simulink model "Full_Motor_Sim"  (R2020b)
settings: Solver=VariableStepAuto  StartTime=0.0  StopTime=1  RelTol=1e-3
libraries: fl_lib x26, ee_lib x20, nesl_utility x19, simulink x12
(part 2 of 2)

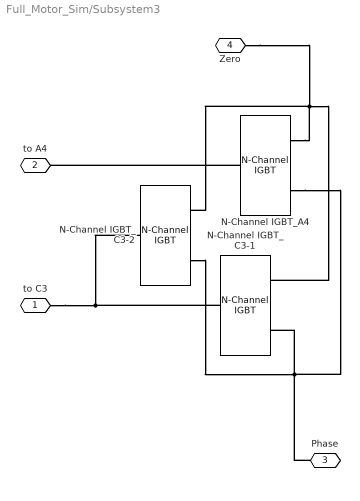
== system Full_Motor_Sim/Subsystem3 ==
  N-Channel IGBT_A4 : ee_lib/Semiconductors & Converters/N-Channel IGBT  model_type=1  Ices=25 uA  Vces=1200 V  Vth=5 V  Vce_sat=1.4 V  Ice_sat=110 A  Vge_sat=15 V  ec=1.3  Tmeas=25 degC  Vge_vec=[ -2 6 7 8 10 12 15 20 ] V  Vce_vec=[ -1 0 0.5 1 1.5 2 2.5 3 3.5 4 ] V  T_vec=[25, 125] degC  Ic_mat=[ -1.015e-5 1.35e-8 4.7135e-4 5.092e-4 5.105e-4 5.117500000000001e-4 5.1299e-4 5.1423e-4 5.1548e-4 5.1672e-4; -9.986899999999999e-6 1.35e-8 4.7135e-4 5.092e-4 5.105e-4 5.117500000000001e-4 5.1299e-4 5.1423e-4 5.1548e-4 5.1672e-4; -9.955e-6 1.35e-8 0.0065225 3.3324 48.154 93.661 105.52 105.72 105.93 106.14; -9.955e-6 1.35e-8 0.0065235 3.5783 70.264 166.33 252.4 317.67 353.38 357.39; -9.955e-6 1.35e-8 0.006524 3.7206 89.17100000000001 228.09 371.63 511.02 642.6900000000001 764.04; -9.9549e-6 1.35e-8 0.0065242 3.7716 97.79300000000001 256.21 424.27 592.92 759.2 921.52; -9.9549e-6 1.35e-8 0.0065243 3.8067 104.52 278.11 464.6 654.37 844.5700000000001 1.0339e+3; -9.9549e-6 1.35e-8 0.0065244 3.8324 109.92 295.67 496.54 702.28 909.96 1.1183e+3 ] A  Ic_mat_3D=zeros(8, 10, 2) A  C_param=3  C_GE=23.7 nF  C_GC=2.7 nF  C_CE=0 nF  C_ies=9.85 nF  C_res=218 pF  C_oes=580 pF  C_GE_vec=[ 25 31 26.5 24.9 25 24.9 24.6 24.7 24.8 ] nF  C_GC_vec=[ 55 9 5.5 3.1 2.5 2.1 1.9 1.8 1.7 ] nF  C_CE_vec=[ 5 11 6.5 4.9 3.5 2.7 2.1 1.7 1.4 ] nF  C_ies_vec=[70 62 60 60 60 60 60 60 60 ] nF  C_res_vec=[ 12 0.46 0.32 0.28 0.24 0.22 0.2 0.19 0.16 ] nF  C_oes_vec=[ 31 0.73 0.515 0.44 0.38 0.34 0.31 0.29 0.28 ] nF  C_Vce_vec=[ 0 5 10 15 20 25 30 35 40 ] V  charge_linearity_param=1  C_OX=20 nF  V_C_OX=-5 V  TF=0 ns  VAF=350 V  RC=0.0001 Ohm  RE=0.0045 Ohm  RG=1 Ohm  BF=100  T_param=2  Ices_T2=620 uA  EG=0.0001 eV  Vce_sat_T2=1.6 V  Tmeas2=150 degC  XTI=1  BEX=-0.6  RG_alpha=1 1/K  Tdevice=150 degC  Tdevice_3D=25 degC  thermal_network_parameterization=ee.enum.thermalNetworkTopology.cauer  Rth=[0, 10] K/W  Rth_Foster=[4, 6] K/W  thermal_mass_parameterization=ee.enum.thermalNetwork.timeconstant  thermal_mass=[0, 1] J/K  thermal_mass_Foster=[1.5, 3] J/K  thermal_time_constant=[0, 10] s  thermal_time_constant_Foster=[6, 18] s  thermal_mass_initial_temperatures=[25, 25] degC  Ic_vec1=[0, 10, 50, 100, 200, 400, 600] A  Vce_vec1=[0, 1.1, 1.3, 1.45, 1.75, 2.25, 2.7] V  Rmiller=0.1 Ohm  Goff=1e-5 1/Ohm  t_on=0.07 us  t_rise=0.7 us  t_off=0.2 us  t_fall=0.5 us  v_meas=300 V  Tj_vec1=[298.15, 398.15] K  Vce_mat1=[0, 1.1, 1.3, 1.45, 1.75, 2.25, 2.7; 0, 1, 1.15, 1.35, 1.7, 2.35, 3] V  E_turn_on_mat1=[0, .2, 1, 2, 4, 8, 15; 0, .3, 1.3, 2.5, 5, 11, 18] * 1e-3 J  E_turn_off_mat1=[0, .3, 1.5, 3, 6, 15, 25; 0, .7, 3.3, 6.5, 13, 25, 35] * 1e-3 J
      settings: SourceProductBaseCode=PS  InternalSimscapePortConfiguration="{\"Bottom\":[],\"Left\":[{\"id\":\"G\",\"label\":\"\",\"type\":\"foundation.electrical.electrical\"}],\"Right\":[{\"id\":\"C\",\"label\":\"\",\"type\":\"foundation.electrical.electrical\"},{\"id\":\"E\",\"label\":\"\",\"type\":\"foundation.electrical.electrical\"}],\"Top\":[]}"
  N-Channel IGBT_C3-1 : ee_lib/Semiconductors & Converters/N-Channel IGBT  model_type=1  Ices=25 uA  Vces=1200 V  Vth=5 V  Vce_sat=2.25 V  Ice_sat=40 A  Vge_sat=7 V  ec=1.5  Tmeas=25 degC  Vge_vec=[ -2 6 7 8 10 12 15 20 ] V  Vce_vec=[ -1 0 0.5 1 1.5 2 2.5 3 3.5 4 ] V  T_vec=[25, 125] degC  Ic_mat=[ -1.015e-5 1.35e-8 4.7135e-4 5.092e-4 5.105e-4 5.117500000000001e-4 5.1299e-4 5.1423e-4 5.1548e-4 5.1672e-4; -9.986899999999999e-6 1.35e-8 4.7135e-4 5.092e-4 5.105e-4 5.117500000000001e-4 5.1299e-4 5.1423e-4 5.1548e-4 5.1672e-4; -9.955e-6 1.35e-8 0.0065225 3.3324 48.154 93.661 105.52 105.72 105.93 106.14; -9.955e-6 1.35e-8 0.0065235 3.5783 70.264 166.33 252.4 317.67 353.38 357.39; -9.955e-6 1.35e-8 0.006524 3.7206 89.17100000000001 228.09 371.63 511.02 642.6900000000001 764.04; -9.9549e-6 1.35e-8 0.0065242 3.7716 97.79300000000001 256.21 424.27 592.92 759.2 921.52; -9.9549e-6 1.35e-8 0.0065243 3.8067 104.52 278.11 464.6 654.37 844.5700000000001 1.0339e+3; -9.9549e-6 1.35e-8 0.0065244 3.8324 109.92 295.67 496.54 702.28 909.96 1.1183e+3 ] A  Ic_mat_3D=zeros(8, 10, 2) A  C_param=3  C_GE=23.7 nF  C_GC=2.7 nF  C_CE=0 nF  C_ies=9.85 nF  C_res=218 pF  C_oes=580 pF  C_GE_vec=[ 25 31 26.5 24.9 25 24.9 24.6 24.7 24.8 ] nF  C_GC_vec=[ 55 9 5.5 3.1 2.5 2.1 1.9 1.8 1.7 ] nF  C_CE_vec=[ 5 11 6.5 4.9 3.5 2.7 2.1 1.7 1.4 ] nF  C_ies_vec=[ 18 13 12 11 10 10 10 10 10 ] nF  C_res_vec=[ 6 2.7 1.9 1.3 0.36 0.22 0.19 0.17 0.16 ] nF  C_oes_vec=[ 8.5 4 3 2 0.8 0.6 0.5 0.48 0.43 ] nF  C_Vce_vec=[ 0 5 10 15 20 25 30 35 40 ] V  charge_linearity_param=1  C_OX=20 nF  V_C_OX=-5 V  TF=0 ns  VAF=10 V  RC=0.005 Ohm  RE=0.009 Ohm  RG=1 kOhm  BF=100  T_param=2  Ices_T2=1.5 mA  EG=0.0001 eV  Vce_sat_T2=2.45 V  Tmeas2=150 degC  XTI=1  BEX=-1  RG_alpha=1 1/K  Tdevice=150 degC  Tdevice_3D=25 degC  thermal_network_parameterization=ee.enum.thermalNetworkTopology.cauer  Rth=[0, 10] K/W  Rth_Foster=[4, 6] K/W  thermal_mass_parameterization=ee.enum.thermalNetwork.timeconstant  thermal_mass=[0, 1] J/K  thermal_mass_Foster=[1.5, 3] J/K  thermal_time_constant=[0, 10] s  thermal_time_constant_Foster=[6, 18] s  thermal_mass_initial_temperatures=[25, 25] degC  Ic_vec1=[0, 10, 50, 100, 200, 400, 600] A  Vce_vec1=[0, 1.1, 1.3, 1.45, 1.75, 2.25, 2.7] V  Rmiller=0.1 Ohm  Goff=1e-5 1/Ohm  t_on=0.07 us  t_rise=0.7 us  t_off=0.2 us  t_fall=0.5 us  v_meas=300 V  Tj_vec1=[298.15, 398.15] K  Vce_mat1=[0, 1.1, 1.3, 1.45, 1.75, 2.25, 2.7; 0, 1, 1.15, 1.35, 1.7, 2.35, 3] V  E_turn_on_mat1=[0, .2, 1, 2, 4, 8, 15; 0, .3, 1.3, 2.5, 5, 11, 18] * 1e-3 J  E_turn_off_mat1=[0, .3, 1.5, 3, 6, 15, 25; 0, .7, 3.3, 6.5, 13, 25, 35] * 1e-3 J
      settings: SourceProductName=Electrical  InternalSimscapePortConfiguration="{\"Bottom\":[],\"Left\":[{\"id\":\"G\",\"label\":\"\",\"type\":\"foundation.electrical.electrical\"}],\"Right\":[{\"id\":\"C\",\"label\":\"\",\"type\":\"foundation.electrical.electrical\"},{\"id\":\"E\",\"label\":\"\",\"type\":\"foundation.electrical.electrical\"}],\"Top\":[]}"
  N-Channel IGBT_C3-2 : ee_lib/Semiconductors & Converters/N-Channel IGBT  model_type=1  Ices=25 uA  Vces=1200 V  Vth=5 V  Vce_sat=2.25 V  Ice_sat=40 A  Vge_sat=7 V  ec=1.5  Tmeas=25 degC  Vge_vec=[ -2 6 7 8 10 12 15 20 ] V  Vce_vec=[ -1 0 0.5 1 1.5 2 2.5 3 3.5 4 ] V  T_vec=[25, 125] degC  Ic_mat=[ -1.015e-5 1.35e-8 4.7135e-4 5.092e-4 5.105e-4 5.117500000000001e-4 5.1299e-4 5.1423e-4 5.1548e-4 5.1672e-4; -9.986899999999999e-6 1.35e-8 4.7135e-4 5.092e-4 5.105e-4 5.117500000000001e-4 5.1299e-4 5.1423e-4 5.1548e-4 5.1672e-4; -9.955e-6 1.35e-8 0.0065225 3.3324 48.154 93.661 105.52 105.72 105.93 106.14; -9.955e-6 1.35e-8 0.0065235 3.5783 70.264 166.33 252.4 317.67 353.38 357.39; -9.955e-6 1.35e-8 0.006524 3.7206 89.17100000000001 228.09 371.63 511.02 642.6900000000001 764.04; -9.9549e-6 1.35e-8 0.0065242 3.7716 97.79300000000001 256.21 424.27 592.92 759.2 921.52; -9.9549e-6 1.35e-8 0.0065243 3.8067 104.52 278.11 464.6 654.37 844.5700000000001 1.0339e+3; -9.9549e-6 1.35e-8 0.0065244 3.8324 109.92 295.67 496.54 702.28 909.96 1.1183e+3 ] A  Ic_mat_3D=zeros(8, 10, 2) A  C_param=3  C_GE=23.7 nF  C_GC=2.7 nF  C_CE=0 nF  C_ies=9.85 nF  C_res=218 pF  C_oes=580 pF  C_GE_vec=[ 25 31 26.5 24.9 25 24.9 24.6 24.7 24.8 ] nF  C_GC_vec=[ 55 9 5.5 3.1 2.5 2.1 1.9 1.8 1.7 ] nF  C_CE_vec=[ 5 11 6.5 4.9 3.5 2.7 2.1 1.7 1.4 ] nF  C_ies_vec=[ 18 13 12 11 10 10 10 10 10 ] nF  C_res_vec=[ 6 2.7 1.9 1.3 0.36 0.22 0.19 0.17 0.16 ] nF  C_oes_vec=[ 8.5 4 3 2 0.8 0.6 0.5 0.48 0.43 ] nF  C_Vce_vec=[ 0 5 10 15 20 25 30 35 40 ] V  charge_linearity_param=1  C_OX=20 nF  V_C_OX=-5 V  TF=0 ns  VAF=10 V  RC=0.005 Ohm  RE=0.009 Ohm  RG=1 kOhm  BF=100  T_param=2  Ices_T2=1.5 mA  EG=0.0001 eV  Vce_sat_T2=2.45 V  Tmeas2=150 degC  XTI=1  BEX=-1  RG_alpha=1 1/K  Tdevice=150 degC  Tdevice_3D=25 degC  thermal_network_parameterization=ee.enum.thermalNetworkTopology.cauer  Rth=[0, 10] K/W  Rth_Foster=[4, 6] K/W  thermal_mass_parameterization=ee.enum.thermalNetwork.timeconstant  thermal_mass=[0, 1] J/K  thermal_mass_Foster=[1.5, 3] J/K  thermal_time_constant=[0, 10] s  thermal_time_constant_Foster=[6, 18] s  thermal_mass_initial_temperatures=[25, 25] degC  Ic_vec1=[0, 10, 50, 100, 200, 400, 600] A  Vce_vec1=[0, 1.1, 1.3, 1.45, 1.75, 2.25, 2.7] V  Rmiller=0.1 Ohm  Goff=1e-5 1/Ohm  t_on=0.07 us  t_rise=0.7 us  t_off=0.2 us  t_fall=0.5 us  v_meas=300 V  Tj_vec1=[298.15, 398.15] K  Vce_mat1=[0, 1.1, 1.3, 1.45, 1.75, 2.25, 2.7; 0, 1, 1.15, 1.35, 1.7, 2.35, 3] V  E_turn_on_mat1=[0, .2, 1, 2, 4, 8, 15; 0, .3, 1.3, 2.5, 5, 11, 18] * 1e-3 J  E_turn_off_mat1=[0, .3, 1.5, 3, 6, 15, 25; 0, .7, 3.3, 6.5, 13, 25, 35] * 1e-3 J
      settings: SourceProductName=Electrical  InternalSimscapePortConfiguration="{\"Bottom\":[],\"Left\":[{\"id\":\"G\",\"label\":\"\",\"type\":\"foundation.electrical.electrical\"}],\"Right\":[{\"id\":\"C\",\"label\":\"\",\"type\":\"foundation.electrical.electrical\"},{\"id\":\"E\",\"label\":\"\",\"type\":\"foundation.electrical.electrical\"}],\"Top\":[]}"
  to C3 : PMIOPort  Side=Left
  to A4 : PMIOPort  Port=2  Side=Left
  Phase : PMIOPort  Port=3  Side=Left
  Zero : PMIOPort  Port=4  Side=Right
  connections:
  N-Channel IGBT_A4/LConn1 -- to A4/RConn1
  Phase/RConn1 -- N-Channel IGBT_C3-2/RConn1 -- N-Channel IGBT_A4/RConn1 -- N-Channel IGBT_C3-1/RConn1
  Zero/RConn1 -- N-Channel IGBT_C3-1/RConn2 -- N-Channel IGBT_A4/RConn2 -- N-Channel IGBT_C3-2/RConn2
  N-Channel IGBT_C3-1/LConn1 -- to C3/RConn1 -- N-Channel IGBT_C3-2/LConn1

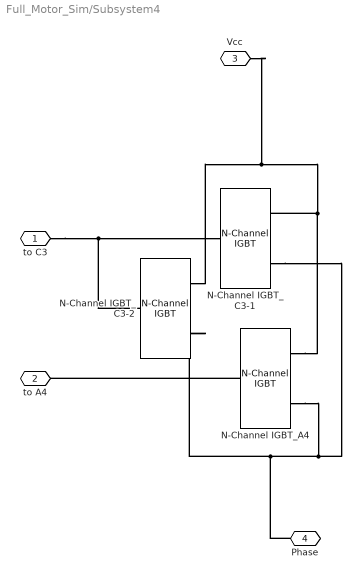
== system Full_Motor_Sim/Subsystem4 ==
  N-Channel IGBT_A4 : ee_lib/Semiconductors & Converters/N-Channel IGBT  model_type=1  Ices=25 uA  Vces=1200 V  Vth=5 V  Vce_sat=1.4 V  Ice_sat=110 A  Vge_sat=15 V  ec=1.3  Tmeas=25 degC  Vge_vec=[ -2 6 7 8 10 12 15 20 ] V  Vce_vec=[ -1 0 0.5 1 1.5 2 2.5 3 3.5 4 ] V  T_vec=[25, 125] degC  Ic_mat=[ -1.015e-5 1.35e-8 4.7135e-4 5.092e-4 5.105e-4 5.117500000000001e-4 5.1299e-4 5.1423e-4 5.1548e-4 5.1672e-4; -9.986899999999999e-6 1.35e-8 4.7135e-4 5.092e-4 5.105e-4 5.117500000000001e-4 5.1299e-4 5.1423e-4 5.1548e-4 5.1672e-4; -9.955e-6 1.35e-8 0.0065225 3.3324 48.154 93.661 105.52 105.72 105.93 106.14; -9.955e-6 1.35e-8 0.0065235 3.5783 70.264 166.33 252.4 317.67 353.38 357.39; -9.955e-6 1.35e-8 0.006524 3.7206 89.17100000000001 228.09 371.63 511.02 642.6900000000001 764.04; -9.9549e-6 1.35e-8 0.0065242 3.7716 97.79300000000001 256.21 424.27 592.92 759.2 921.52; -9.9549e-6 1.35e-8 0.0065243 3.8067 104.52 278.11 464.6 654.37 844.5700000000001 1.0339e+3; -9.9549e-6 1.35e-8 0.0065244 3.8324 109.92 295.67 496.54 702.28 909.96 1.1183e+3 ] A  Ic_mat_3D=zeros(8, 10, 2) A  C_param=3  C_GE=23.7 nF  C_GC=2.7 nF  C_CE=0 nF  C_ies=9.85 nF  C_res=218 pF  C_oes=580 pF  C_GE_vec=[ 25 31 26.5 24.9 25 24.9 24.6 24.7 24.8 ] nF  C_GC_vec=[ 55 9 5.5 3.1 2.5 2.1 1.9 1.8 1.7 ] nF  C_CE_vec=[ 5 11 6.5 4.9 3.5 2.7 2.1 1.7 1.4 ] nF  C_ies_vec=[70 62 60 60 60 60 60 60 60 ] nF  C_res_vec=[ 12 0.46 0.32 0.28 0.24 0.22 0.2 0.19 0.16 ] nF  C_oes_vec=[ 31 0.73 0.515 0.44 0.38 0.34 0.31 0.29 0.28 ] nF  C_Vce_vec=[ 0 5 10 15 20 25 30 35 40 ] V  charge_linearity_param=1  C_OX=20 nF  V_C_OX=-5 V  TF=0 ns  VAF=350 V  RC=0.0001 Ohm  RE=0.0045 Ohm  RG=1 Ohm  BF=100  T_param=2  Ices_T2=620 uA  EG=0.0001 eV  Vce_sat_T2=1.6 V  Tmeas2=150 degC  XTI=1  BEX=-0.6  RG_alpha=1 1/K  Tdevice=150 degC  Tdevice_3D=25 degC  thermal_network_parameterization=ee.enum.thermalNetworkTopology.cauer  Rth=[0, 10] K/W  Rth_Foster=[4, 6] K/W  thermal_mass_parameterization=ee.enum.thermalNetwork.timeconstant  thermal_mass=[0, 1] J/K  thermal_mass_Foster=[1.5, 3] J/K  thermal_time_constant=[0, 10] s  thermal_time_constant_Foster=[6, 18] s  thermal_mass_initial_temperatures=[25, 25] degC  Ic_vec1=[0, 10, 50, 100, 200, 400, 600] A  Vce_vec1=[0, 1.1, 1.3, 1.45, 1.75, 2.25, 2.7] V  Rmiller=0.1 Ohm  Goff=1e-5 1/Ohm  t_on=0.07 us  t_rise=0.7 us  t_off=0.2 us  t_fall=0.5 us  v_meas=300 V  Tj_vec1=[298.15, 398.15] K  Vce_mat1=[0, 1.1, 1.3, 1.45, 1.75, 2.25, 2.7; 0, 1, 1.15, 1.35, 1.7, 2.35, 3] V  E_turn_on_mat1=[0, .2, 1, 2, 4, 8, 15; 0, .3, 1.3, 2.5, 5, 11, 18] * 1e-3 J  E_turn_off_mat1=[0, .3, 1.5, 3, 6, 15, 25; 0, .7, 3.3, 6.5, 13, 25, 35] * 1e-3 J
      settings: SourceProductBaseCode=PS  InternalSimscapePortConfiguration="{\"Bottom\":[],\"Left\":[{\"id\":\"G\",\"label\":\"\",\"type\":\"foundation.electrical.electrical\"}],\"Right\":[{\"id\":\"C\",\"label\":\"\",\"type\":\"foundation.electrical.electrical\"},{\"id\":\"E\",\"label\":\"\",\"type\":\"foundation.electrical.electrical\"}],\"Top\":[]}"
  N-Channel IGBT_C3-1 : ee_lib/Semiconductors & Converters/N-Channel IGBT  model_type=1  Ices=25 uA  Vces=1200 V  Vth=5 V  Vce_sat=2.25 V  Ice_sat=40 A  Vge_sat=7 V  ec=1.5  Tmeas=25 degC  Vge_vec=[ -2 6 7 8 10 12 15 20 ] V  Vce_vec=[ -1 0 0.5 1 1.5 2 2.5 3 3.5 4 ] V  T_vec=[25, 125] degC  Ic_mat=[ -1.015e-5 1.35e-8 4.7135e-4 5.092e-4 5.105e-4 5.117500000000001e-4 5.1299e-4 5.1423e-4 5.1548e-4 5.1672e-4; -9.986899999999999e-6 1.35e-8 4.7135e-4 5.092e-4 5.105e-4 5.117500000000001e-4 5.1299e-4 5.1423e-4 5.1548e-4 5.1672e-4; -9.955e-6 1.35e-8 0.0065225 3.3324 48.154 93.661 105.52 105.72 105.93 106.14; -9.955e-6 1.35e-8 0.0065235 3.5783 70.264 166.33 252.4 317.67 353.38 357.39; -9.955e-6 1.35e-8 0.006524 3.7206 89.17100000000001 228.09 371.63 511.02 642.6900000000001 764.04; -9.9549e-6 1.35e-8 0.0065242 3.7716 97.79300000000001 256.21 424.27 592.92 759.2 921.52; -9.9549e-6 1.35e-8 0.0065243 3.8067 104.52 278.11 464.6 654.37 844.5700000000001 1.0339e+3; -9.9549e-6 1.35e-8 0.0065244 3.8324 109.92 295.67 496.54 702.28 909.96 1.1183e+3 ] A  Ic_mat_3D=zeros(8, 10, 2) A  C_param=3  C_GE=23.7 nF  C_GC=2.7 nF  C_CE=0 nF  C_ies=9.85 nF  C_res=218 pF  C_oes=580 pF  C_GE_vec=[ 25 31 26.5 24.9 25 24.9 24.6 24.7 24.8 ] nF  C_GC_vec=[ 55 9 5.5 3.1 2.5 2.1 1.9 1.8 1.7 ] nF  C_CE_vec=[ 5 11 6.5 4.9 3.5 2.7 2.1 1.7 1.4 ] nF  C_ies_vec=[ 18 13 12 11 10 10 10 10 10 ] nF  C_res_vec=[ 6 2.7 1.9 1.3 0.36 0.22 0.19 0.17 0.16 ] nF  C_oes_vec=[ 8.5 4 3 2 0.8 0.6 0.5 0.48 0.43 ] nF  C_Vce_vec=[ 0 5 10 15 20 25 30 35 40 ] V  charge_linearity_param=1  C_OX=20 nF  V_C_OX=-5 V  TF=0 ns  VAF=10 V  RC=0.005 Ohm  RE=0.009 Ohm  RG=1 kOhm  BF=100  T_param=2  Ices_T2=1.5 mA  EG=0.0001 eV  Vce_sat_T2=2.45 V  Tmeas2=150 degC  XTI=1  BEX=-1  RG_alpha=1 1/K  Tdevice=150 degC  Tdevice_3D=25 degC  thermal_network_parameterization=ee.enum.thermalNetworkTopology.cauer  Rth=[0, 10] K/W  Rth_Foster=[4, 6] K/W  thermal_mass_parameterization=ee.enum.thermalNetwork.timeconstant  thermal_mass=[0, 1] J/K  thermal_mass_Foster=[1.5, 3] J/K  thermal_time_constant=[0, 10] s  thermal_time_constant_Foster=[6, 18] s  thermal_mass_initial_temperatures=[25, 25] degC  Ic_vec1=[0, 10, 50, 100, 200, 400, 600] A  Vce_vec1=[0, 1.1, 1.3, 1.45, 1.75, 2.25, 2.7] V  Rmiller=0.1 Ohm  Goff=1e-5 1/Ohm  t_on=0.07 us  t_rise=0.7 us  t_off=0.2 us  t_fall=0.5 us  v_meas=300 V  Tj_vec1=[298.15, 398.15] K  Vce_mat1=[0, 1.1, 1.3, 1.45, 1.75, 2.25, 2.7; 0, 1, 1.15, 1.35, 1.7, 2.35, 3] V  E_turn_on_mat1=[0, .2, 1, 2, 4, 8, 15; 0, .3, 1.3, 2.5, 5, 11, 18] * 1e-3 J  E_turn_off_mat1=[0, .3, 1.5, 3, 6, 15, 25; 0, .7, 3.3, 6.5, 13, 25, 35] * 1e-3 J
      settings: SourceProductName=Electrical  InternalSimscapePortConfiguration="{\"Bottom\":[],\"Left\":[{\"id\":\"G\",\"label\":\"\",\"type\":\"foundation.electrical.electrical\"}],\"Right\":[{\"id\":\"C\",\"label\":\"\",\"type\":\"foundation.electrical.electrical\"},{\"id\":\"E\",\"label\":\"\",\"type\":\"foundation.electrical.electrical\"}],\"Top\":[]}"
  N-Channel IGBT_C3-2 : ee_lib/Semiconductors & Converters/N-Channel IGBT  model_type=1  Ices=25 uA  Vces=1200 V  Vth=5 V  Vce_sat=2.25 V  Ice_sat=40 A  Vge_sat=7 V  ec=1.5  Tmeas=25 degC  Vge_vec=[ -2 6 7 8 10 12 15 20 ] V  Vce_vec=[ -1 0 0.5 1 1.5 2 2.5 3 3.5 4 ] V  T_vec=[25, 125] degC  Ic_mat=[ -1.015e-5 1.35e-8 4.7135e-4 5.092e-4 5.105e-4 5.117500000000001e-4 5.1299e-4 5.1423e-4 5.1548e-4 5.1672e-4; -9.986899999999999e-6 1.35e-8 4.7135e-4 5.092e-4 5.105e-4 5.117500000000001e-4 5.1299e-4 5.1423e-4 5.1548e-4 5.1672e-4; -9.955e-6 1.35e-8 0.0065225 3.3324 48.154 93.661 105.52 105.72 105.93 106.14; -9.955e-6 1.35e-8 0.0065235 3.5783 70.264 166.33 252.4 317.67 353.38 357.39; -9.955e-6 1.35e-8 0.006524 3.7206 89.17100000000001 228.09 371.63 511.02 642.6900000000001 764.04; -9.9549e-6 1.35e-8 0.0065242 3.7716 97.79300000000001 256.21 424.27 592.92 759.2 921.52; -9.9549e-6 1.35e-8 0.0065243 3.8067 104.52 278.11 464.6 654.37 844.5700000000001 1.0339e+3; -9.9549e-6 1.35e-8 0.0065244 3.8324 109.92 295.67 496.54 702.28 909.96 1.1183e+3 ] A  Ic_mat_3D=zeros(8, 10, 2) A  C_param=3  C_GE=23.7 nF  C_GC=2.7 nF  C_CE=0 nF  C_ies=9.85 nF  C_res=218 pF  C_oes=580 pF  C_GE_vec=[ 25 31 26.5 24.9 25 24.9 24.6 24.7 24.8 ] nF  C_GC_vec=[ 55 9 5.5 3.1 2.5 2.1 1.9 1.8 1.7 ] nF  C_CE_vec=[ 5 11 6.5 4.9 3.5 2.7 2.1 1.7 1.4 ] nF  C_ies_vec=[ 18 13 12 11 10 10 10 10 10 ] nF  C_res_vec=[ 6 2.7 1.9 1.3 0.36 0.22 0.19 0.17 0.16 ] nF  C_oes_vec=[ 8.5 4 3 2 0.8 0.6 0.5 0.48 0.43 ] nF  C_Vce_vec=[ 0 5 10 15 20 25 30 35 40 ] V  charge_linearity_param=1  C_OX=20 nF  V_C_OX=-5 V  TF=0 ns  VAF=10 V  RC=0.005 Ohm  RE=0.009 Ohm  RG=1 kOhm  BF=100  T_param=2  Ices_T2=1.5 mA  EG=0.0001 eV  Vce_sat_T2=2.45 V  Tmeas2=150 degC  XTI=1  BEX=-1  RG_alpha=1 1/K  Tdevice=150 degC  Tdevice_3D=25 degC  thermal_network_parameterization=ee.enum.thermalNetworkTopology.cauer  Rth=[0, 10] K/W  Rth_Foster=[4, 6] K/W  thermal_mass_parameterization=ee.enum.thermalNetwork.timeconstant  thermal_mass=[0, 1] J/K  thermal_mass_Foster=[1.5, 3] J/K  thermal_time_constant=[0, 10] s  thermal_time_constant_Foster=[6, 18] s  thermal_mass_initial_temperatures=[25, 25] degC  Ic_vec1=[0, 10, 50, 100, 200, 400, 600] A  Vce_vec1=[0, 1.1, 1.3, 1.45, 1.75, 2.25, 2.7] V  Rmiller=0.1 Ohm  Goff=1e-5 1/Ohm  t_on=0.07 us  t_rise=0.7 us  t_off=0.2 us  t_fall=0.5 us  v_meas=300 V  Tj_vec1=[298.15, 398.15] K  Vce_mat1=[0, 1.1, 1.3, 1.45, 1.75, 2.25, 2.7; 0, 1, 1.15, 1.35, 1.7, 2.35, 3] V  E_turn_on_mat1=[0, .2, 1, 2, 4, 8, 15; 0, .3, 1.3, 2.5, 5, 11, 18] * 1e-3 J  E_turn_off_mat1=[0, .3, 1.5, 3, 6, 15, 25; 0, .7, 3.3, 6.5, 13, 25, 35] * 1e-3 J
      settings: SourceProductName=Electrical  InternalSimscapePortConfiguration="{\"Bottom\":[],\"Left\":[{\"id\":\"G\",\"label\":\"\",\"type\":\"foundation.electrical.electrical\"}],\"Right\":[{\"id\":\"C\",\"label\":\"\",\"type\":\"foundation.electrical.electrical\"},{\"id\":\"E\",\"label\":\"\",\"type\":\"foundation.electrical.electrical\"}],\"Top\":[]}"
  to C3 : PMIOPort  Side=Left
  to A4 : PMIOPort  Port=2  Side=Left
  Vcc : PMIOPort  Port=3  Side=Left
  Phase : PMIOPort  Port=4  Side=Right
  connections:
  N-Channel IGBT_C3-1/RConn1 -- N-Channel IGBT_A4/RConn1 -- N-Channel IGBT_C3-2/RConn1 -- Vcc/RConn1
  N-Channel IGBT_C3-2/RConn2 -- N-Channel IGBT_C3-1/RConn2 -- N-Channel IGBT_A4/RConn2 -- Phase/RConn1
  N-Channel IGBT_C3-1/LConn1 -- to C3/RConn1 -- N-Channel IGBT_C3-2/LConn1
  N-Channel IGBT_A4/LConn1 -- to A4/RConn1

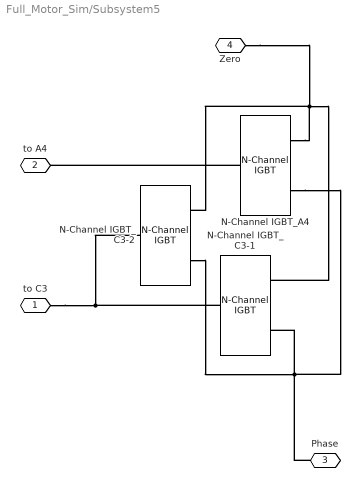
== system Full_Motor_Sim/Subsystem5 ==
  N-Channel IGBT_A4 : ee_lib/Semiconductors & Converters/N-Channel IGBT  model_type=1  Ices=25 uA  Vces=1200 V  Vth=5 V  Vce_sat=1.4 V  Ice_sat=110 A  Vge_sat=15 V  ec=1.3  Tmeas=25 degC  Vge_vec=[ -2 6 7 8 10 12 15 20 ] V  Vce_vec=[ -1 0 0.5 1 1.5 2 2.5 3 3.5 4 ] V  T_vec=[25, 125] degC  Ic_mat=[ -1.015e-5 1.35e-8 4.7135e-4 5.092e-4 5.105e-4 5.117500000000001e-4 5.1299e-4 5.1423e-4 5.1548e-4 5.1672e-4; -9.986899999999999e-6 1.35e-8 4.7135e-4 5.092e-4 5.105e-4 5.117500000000001e-4 5.1299e-4 5.1423e-4 5.1548e-4 5.1672e-4; -9.955e-6 1.35e-8 0.0065225 3.3324 48.154 93.661 105.52 105.72 105.93 106.14; -9.955e-6 1.35e-8 0.0065235 3.5783 70.264 166.33 252.4 317.67 353.38 357.39; -9.955e-6 1.35e-8 0.006524 3.7206 89.17100000000001 228.09 371.63 511.02 642.6900000000001 764.04; -9.9549e-6 1.35e-8 0.0065242 3.7716 97.79300000000001 256.21 424.27 592.92 759.2 921.52; -9.9549e-6 1.35e-8 0.0065243 3.8067 104.52 278.11 464.6 654.37 844.5700000000001 1.0339e+3; -9.9549e-6 1.35e-8 0.0065244 3.8324 109.92 295.67 496.54 702.28 909.96 1.1183e+3 ] A  Ic_mat_3D=zeros(8, 10, 2) A  C_param=3  C_GE=23.7 nF  C_GC=2.7 nF  C_CE=0 nF  C_ies=9.85 nF  C_res=218 pF  C_oes=580 pF  C_GE_vec=[ 25 31 26.5 24.9 25 24.9 24.6 24.7 24.8 ] nF  C_GC_vec=[ 55 9 5.5 3.1 2.5 2.1 1.9 1.8 1.7 ] nF  C_CE_vec=[ 5 11 6.5 4.9 3.5 2.7 2.1 1.7 1.4 ] nF  C_ies_vec=[70 62 60 60 60 60 60 60 60 ] nF  C_res_vec=[ 12 0.46 0.32 0.28 0.24 0.22 0.2 0.19 0.16 ] nF  C_oes_vec=[ 31 0.73 0.515 0.44 0.38 0.34 0.31 0.29 0.28 ] nF  C_Vce_vec=[ 0 5 10 15 20 25 30 35 40 ] V  charge_linearity_param=1  C_OX=20 nF  V_C_OX=-5 V  TF=0 ns  VAF=350 V  RC=0.0001 Ohm  RE=0.0045 Ohm  RG=1 Ohm  BF=100  T_param=2  Ices_T2=620 uA  EG=0.0001 eV  Vce_sat_T2=1.6 V  Tmeas2=150 degC  XTI=1  BEX=-0.6  RG_alpha=1 1/K  Tdevice=150 degC  Tdevice_3D=25 degC  thermal_network_parameterization=ee.enum.thermalNetworkTopology.cauer  Rth=[0, 10] K/W  Rth_Foster=[4, 6] K/W  thermal_mass_parameterization=ee.enum.thermalNetwork.timeconstant  thermal_mass=[0, 1] J/K  thermal_mass_Foster=[1.5, 3] J/K  thermal_time_constant=[0, 10] s  thermal_time_constant_Foster=[6, 18] s  thermal_mass_initial_temperatures=[25, 25] degC  Ic_vec1=[0, 10, 50, 100, 200, 400, 600] A  Vce_vec1=[0, 1.1, 1.3, 1.45, 1.75, 2.25, 2.7] V  Rmiller=0.1 Ohm  Goff=1e-5 1/Ohm  t_on=0.07 us  t_rise=0.7 us  t_off=0.2 us  t_fall=0.5 us  v_meas=300 V  Tj_vec1=[298.15, 398.15] K  Vce_mat1=[0, 1.1, 1.3, 1.45, 1.75, 2.25, 2.7; 0, 1, 1.15, 1.35, 1.7, 2.35, 3] V  E_turn_on_mat1=[0, .2, 1, 2, 4, 8, 15; 0, .3, 1.3, 2.5, 5, 11, 18] * 1e-3 J  E_turn_off_mat1=[0, .3, 1.5, 3, 6, 15, 25; 0, .7, 3.3, 6.5, 13, 25, 35] * 1e-3 J
      settings: SourceProductBaseCode=PS  InternalSimscapePortConfiguration="{\"Bottom\":[],\"Left\":[{\"id\":\"G\",\"label\":\"\",\"type\":\"foundation.electrical.electrical\"}],\"Right\":[{\"id\":\"C\",\"label\":\"\",\"type\":\"foundation.electrical.electrical\"},{\"id\":\"E\",\"label\":\"\",\"type\":\"foundation.electrical.electrical\"}],\"Top\":[]}"
  N-Channel IGBT_C3-1 : ee_lib/Semiconductors & Converters/N-Channel IGBT  model_type=1  Ices=25 uA  Vces=1200 V  Vth=5 V  Vce_sat=2.25 V  Ice_sat=40 A  Vge_sat=7 V  ec=1.5  Tmeas=25 degC  Vge_vec=[ -2 6 7 8 10 12 15 20 ] V  Vce_vec=[ -1 0 0.5 1 1.5 2 2.5 3 3.5 4 ] V  T_vec=[25, 125] degC  Ic_mat=[ -1.015e-5 1.35e-8 4.7135e-4 5.092e-4 5.105e-4 5.117500000000001e-4 5.1299e-4 5.1423e-4 5.1548e-4 5.1672e-4; -9.986899999999999e-6 1.35e-8 4.7135e-4 5.092e-4 5.105e-4 5.117500000000001e-4 5.1299e-4 5.1423e-4 5.1548e-4 5.1672e-4; -9.955e-6 1.35e-8 0.0065225 3.3324 48.154 93.661 105.52 105.72 105.93 106.14; -9.955e-6 1.35e-8 0.0065235 3.5783 70.264 166.33 252.4 317.67 353.38 357.39; -9.955e-6 1.35e-8 0.006524 3.7206 89.17100000000001 228.09 371.63 511.02 642.6900000000001 764.04; -9.9549e-6 1.35e-8 0.0065242 3.7716 97.79300000000001 256.21 424.27 592.92 759.2 921.52; -9.9549e-6 1.35e-8 0.0065243 3.8067 104.52 278.11 464.6 654.37 844.5700000000001 1.0339e+3; -9.9549e-6 1.35e-8 0.0065244 3.8324 109.92 295.67 496.54 702.28 909.96 1.1183e+3 ] A  Ic_mat_3D=zeros(8, 10, 2) A  C_param=3  C_GE=23.7 nF  C_GC=2.7 nF  C_CE=0 nF  C_ies=9.85 nF  C_res=218 pF  C_oes=580 pF  C_GE_vec=[ 25 31 26.5 24.9 25 24.9 24.6 24.7 24.8 ] nF  C_GC_vec=[ 55 9 5.5 3.1 2.5 2.1 1.9 1.8 1.7 ] nF  C_CE_vec=[ 5 11 6.5 4.9 3.5 2.7 2.1 1.7 1.4 ] nF  C_ies_vec=[ 18 13 12 11 10 10 10 10 10 ] nF  C_res_vec=[ 6 2.7 1.9 1.3 0.36 0.22 0.19 0.17 0.16 ] nF  C_oes_vec=[ 8.5 4 3 2 0.8 0.6 0.5 0.48 0.43 ] nF  C_Vce_vec=[ 0 5 10 15 20 25 30 35 40 ] V  charge_linearity_param=1  C_OX=20 nF  V_C_OX=-5 V  TF=0 ns  VAF=10 V  RC=0.005 Ohm  RE=0.009 Ohm  RG=1 kOhm  BF=100  T_param=2  Ices_T2=1.5 mA  EG=0.0001 eV  Vce_sat_T2=2.45 V  Tmeas2=150 degC  XTI=1  BEX=-1  RG_alpha=1 1/K  Tdevice=150 degC  Tdevice_3D=25 degC  thermal_network_parameterization=ee.enum.thermalNetworkTopology.cauer  Rth=[0, 10] K/W  Rth_Foster=[4, 6] K/W  thermal_mass_parameterization=ee.enum.thermalNetwork.timeconstant  thermal_mass=[0, 1] J/K  thermal_mass_Foster=[1.5, 3] J/K  thermal_time_constant=[0, 10] s  thermal_time_constant_Foster=[6, 18] s  thermal_mass_initial_temperatures=[25, 25] degC  Ic_vec1=[0, 10, 50, 100, 200, 400, 600] A  Vce_vec1=[0, 1.1, 1.3, 1.45, 1.75, 2.25, 2.7] V  Rmiller=0.1 Ohm  Goff=1e-5 1/Ohm  t_on=0.07 us  t_rise=0.7 us  t_off=0.2 us  t_fall=0.5 us  v_meas=300 V  Tj_vec1=[298.15, 398.15] K  Vce_mat1=[0, 1.1, 1.3, 1.45, 1.75, 2.25, 2.7; 0, 1, 1.15, 1.35, 1.7, 2.35, 3] V  E_turn_on_mat1=[0, .2, 1, 2, 4, 8, 15; 0, .3, 1.3, 2.5, 5, 11, 18] * 1e-3 J  E_turn_off_mat1=[0, .3, 1.5, 3, 6, 15, 25; 0, .7, 3.3, 6.5, 13, 25, 35] * 1e-3 J
      settings: SourceProductName=Electrical  InternalSimscapePortConfiguration="{\"Bottom\":[],\"Left\":[{\"id\":\"G\",\"label\":\"\",\"type\":\"foundation.electrical.electrical\"}],\"Right\":[{\"id\":\"C\",\"label\":\"\",\"type\":\"foundation.electrical.electrical\"},{\"id\":\"E\",\"label\":\"\",\"type\":\"foundation.electrical.electrical\"}],\"Top\":[]}"
  N-Channel IGBT_C3-2 : ee_lib/Semiconductors & Converters/N-Channel IGBT  model_type=1  Ices=25 uA  Vces=1200 V  Vth=5 V  Vce_sat=2.25 V  Ice_sat=40 A  Vge_sat=7 V  ec=1.5  Tmeas=25 degC  Vge_vec=[ -2 6 7 8 10 12 15 20 ] V  Vce_vec=[ -1 0 0.5 1 1.5 2 2.5 3 3.5 4 ] V  T_vec=[25, 125] degC  Ic_mat=[ -1.015e-5 1.35e-8 4.7135e-4 5.092e-4 5.105e-4 5.117500000000001e-4 5.1299e-4 5.1423e-4 5.1548e-4 5.1672e-4; -9.986899999999999e-6 1.35e-8 4.7135e-4 5.092e-4 5.105e-4 5.117500000000001e-4 5.1299e-4 5.1423e-4 5.1548e-4 5.1672e-4; -9.955e-6 1.35e-8 0.0065225 3.3324 48.154 93.661 105.52 105.72 105.93 106.14; -9.955e-6 1.35e-8 0.0065235 3.5783 70.264 166.33 252.4 317.67 353.38 357.39; -9.955e-6 1.35e-8 0.006524 3.7206 89.17100000000001 228.09 371.63 511.02 642.6900000000001 764.04; -9.9549e-6 1.35e-8 0.0065242 3.7716 97.79300000000001 256.21 424.27 592.92 759.2 921.52; -9.9549e-6 1.35e-8 0.0065243 3.8067 104.52 278.11 464.6 654.37 844.5700000000001 1.0339e+3; -9.9549e-6 1.35e-8 0.0065244 3.8324 109.92 295.67 496.54 702.28 909.96 1.1183e+3 ] A  Ic_mat_3D=zeros(8, 10, 2) A  C_param=3  C_GE=23.7 nF  C_GC=2.7 nF  C_CE=0 nF  C_ies=9.85 nF  C_res=218 pF  C_oes=580 pF  C_GE_vec=[ 25 31 26.5 24.9 25 24.9 24.6 24.7 24.8 ] nF  C_GC_vec=[ 55 9 5.5 3.1 2.5 2.1 1.9 1.8 1.7 ] nF  C_CE_vec=[ 5 11 6.5 4.9 3.5 2.7 2.1 1.7 1.4 ] nF  C_ies_vec=[ 18 13 12 11 10 10 10 10 10 ] nF  C_res_vec=[ 6 2.7 1.9 1.3 0.36 0.22 0.19 0.17 0.16 ] nF  C_oes_vec=[ 8.5 4 3 2 0.8 0.6 0.5 0.48 0.43 ] nF  C_Vce_vec=[ 0 5 10 15 20 25 30 35 40 ] V  charge_linearity_param=1  C_OX=20 nF  V_C_OX=-5 V  TF=0 ns  VAF=10 V  RC=0.005 Ohm  RE=0.009 Ohm  RG=1 kOhm  BF=100  T_param=2  Ices_T2=1.5 mA  EG=0.0001 eV  Vce_sat_T2=2.45 V  Tmeas2=150 degC  XTI=1  BEX=-1  RG_alpha=1 1/K  Tdevice=150 degC  Tdevice_3D=25 degC  thermal_network_parameterization=ee.enum.thermalNetworkTopology.cauer  Rth=[0, 10] K/W  Rth_Foster=[4, 6] K/W  thermal_mass_parameterization=ee.enum.thermalNetwork.timeconstant  thermal_mass=[0, 1] J/K  thermal_mass_Foster=[1.5, 3] J/K  thermal_time_constant=[0, 10] s  thermal_time_constant_Foster=[6, 18] s  thermal_mass_initial_temperatures=[25, 25] degC  Ic_vec1=[0, 10, 50, 100, 200, 400, 600] A  Vce_vec1=[0, 1.1, 1.3, 1.45, 1.75, 2.25, 2.7] V  Rmiller=0.1 Ohm  Goff=1e-5 1/Ohm  t_on=0.07 us  t_rise=0.7 us  t_off=0.2 us  t_fall=0.5 us  v_meas=300 V  Tj_vec1=[298.15, 398.15] K  Vce_mat1=[0, 1.1, 1.3, 1.45, 1.75, 2.25, 2.7; 0, 1, 1.15, 1.35, 1.7, 2.35, 3] V  E_turn_on_mat1=[0, .2, 1, 2, 4, 8, 15; 0, .3, 1.3, 2.5, 5, 11, 18] * 1e-3 J  E_turn_off_mat1=[0, .3, 1.5, 3, 6, 15, 25; 0, .7, 3.3, 6.5, 13, 25, 35] * 1e-3 J
      settings: SourceProductName=Electrical  InternalSimscapePortConfiguration="{\"Bottom\":[],\"Left\":[{\"id\":\"G\",\"label\":\"\",\"type\":\"foundation.electrical.electrical\"}],\"Right\":[{\"id\":\"C\",\"label\":\"\",\"type\":\"foundation.electrical.electrical\"},{\"id\":\"E\",\"label\":\"\",\"type\":\"foundation.electrical.electrical\"}],\"Top\":[]}"
  to C3 : PMIOPort  Side=Left
  to A4 : PMIOPort  Port=2  Side=Left
  Phase : PMIOPort  Port=3  Side=Left
  Zero : PMIOPort  Port=4  Side=Right
  connections:
  N-Channel IGBT_C3-2/LConn1 -- to C3/RConn1 -- N-Channel IGBT_C3-1/LConn1
  N-Channel IGBT_C3-2/RConn2 -- N-Channel IGBT_A4/RConn2 -- N-Channel IGBT_C3-1/RConn2 -- Zero/RConn1
  N-Channel IGBT_C3-1/RConn1 -- N-Channel IGBT_A4/RConn1 -- N-Channel IGBT_C3-2/RConn1 -- Phase/RConn1
  N-Channel IGBT_A4/LConn1 -- to A4/RConn1

== system Full_Motor_Sim/Subsystem6 ==
  N-Channel IGBT_A4 : ee_lib/Semiconductors & Converters/N-Channel IGBT  model_type=1  Ices=25 uA  Vces=1200 V  Vth=5 V  Vce_sat=1.4 V  Ice_sat=110 A  Vge_sat=15 V  ec=1.3  Tmeas=25 degC  Vge_vec=[ -2 6 7 8 10 12 15 20 ] V  Vce_vec=[ -1 0 0.5 1 1.5 2 2.5 3 3.5 4 ] V  T_vec=[25, 125] degC  Ic_mat=[ -1.015e-5 1.35e-8 4.7135e-4 5.092e-4 5.105e-4 5.117500000000001e-4 5.1299e-4 5.1423e-4 5.1548e-4 5.1672e-4; -9.986899999999999e-6 1.35e-8 4.7135e-4 5.092e-4 5.105e-4 5.117500000000001e-4 5.1299e-4 5.1423e-4 5.1548e-4 5.1672e-4; -9.955e-6 1.35e-8 0.0065225 3.3324 48.154 93.661 105.52 105.72 105.93 106.14; -9.955e-6 1.35e-8 0.0065235 3.5783 70.264 166.33 252.4 317.67 353.38 357.39; -9.955e-6 1.35e-8 0.006524 3.7206 89.17100000000001 228.09 371.63 511.02 642.6900000000001 764.04; -9.9549e-6 1.35e-8 0.0065242 3.7716 97.79300000000001 256.21 424.27 592.92 759.2 921.52; -9.9549e-6 1.35e-8 0.0065243 3.8067 104.52 278.11 464.6 654.37 844.5700000000001 1.0339e+3; -9.9549e-6 1.35e-8 0.0065244 3.8324 109.92 295.67 496.54 702.28 909.96 1.1183e+3 ] A  Ic_mat_3D=zeros(8, 10, 2) A  C_param=3  C_GE=23.7 nF  C_GC=2.7 nF  C_CE=0 nF  C_ies=9.85 nF  C_res=218 pF  C_oes=580 pF  C_GE_vec=[ 25 31 26.5 24.9 25 24.9 24.6 24.7 24.8 ] nF  C_GC_vec=[ 55 9 5.5 3.1 2.5 2.1 1.9 1.8 1.7 ] nF  C_CE_vec=[ 5 11 6.5 4.9 3.5 2.7 2.1 1.7 1.4 ] nF  C_ies_vec=[70 62 60 60 60 60 60 60 60 ] nF  C_res_vec=[ 12 0.46 0.32 0.28 0.24 0.22 0.2 0.19 0.16 ] nF  C_oes_vec=[ 31 0.73 0.515 0.44 0.38 0.34 0.31 0.29 0.28 ] nF  C_Vce_vec=[ 0 5 10 15 20 25 30 35 40 ] V  charge_linearity_param=1  C_OX=20 nF  V_C_OX=-5 V  TF=0 ns  VAF=350 V  RC=0.0001 Ohm  RE=0.0045 Ohm  RG=1 Ohm  BF=100  T_param=2  Ices_T2=620 uA  EG=0.0001 eV  Vce_sat_T2=1.6 V  Tmeas2=150 degC  XTI=1  BEX=-0.6  RG_alpha=1 1/K  Tdevice=150 degC  Tdevice_3D=25 degC  thermal_network_parameterization=ee.enum.thermalNetworkTopology.cauer  Rth=[0, 10] K/W  Rth_Foster=[4, 6] K/W  thermal_mass_parameterization=ee.enum.thermalNetwork.timeconstant  thermal_mass=[0, 1] J/K  thermal_mass_Foster=[1.5, 3] J/K  thermal_time_constant=[0, 10] s  thermal_time_constant_Foster=[6, 18] s  thermal_mass_initial_temperatures=[25, 25] degC  Ic_vec1=[0, 10, 50, 100, 200, 400, 600] A  Vce_vec1=[0, 1.1, 1.3, 1.45, 1.75, 2.25, 2.7] V  Rmiller=0.1 Ohm  Goff=1e-5 1/Ohm  t_on=0.07 us  t_rise=0.7 us  t_off=0.2 us  t_fall=0.5 us  v_meas=300 V  Tj_vec1=[298.15, 398.15] K  Vce_mat1=[0, 1.1, 1.3, 1.45, 1.75, 2.25, 2.7; 0, 1, 1.15, 1.35, 1.7, 2.35, 3] V  E_turn_on_mat1=[0, .2, 1, 2, 4, 8, 15; 0, .3, 1.3, 2.5, 5, 11, 18] * 1e-3 J  E_turn_off_mat1=[0, .3, 1.5, 3, 6, 15, 25; 0, .7, 3.3, 6.5, 13, 25, 35] * 1e-3 J
      settings: SourceProductBaseCode=PS  InternalSimscapePortConfiguration="{\"Bottom\":[],\"Left\":[{\"id\":\"G\",\"label\":\"\",\"type\":\"foundation.electrical.electrical\"}],\"Right\":[{\"id\":\"C\",\"label\":\"\",\"type\":\"foundation.electrical.electrical\"},{\"id\":\"E\",\"label\":\"\",\"type\":\"foundation.electrical.electrical\"}],\"Top\":[]}"
  N-Channel IGBT_C3-1 : ee_lib/Semiconductors & Converters/N-Channel IGBT  model_type=1  Ices=25 uA  Vces=1200 V  Vth=5 V  Vce_sat=2.25 V  Ice_sat=40 A  Vge_sat=7 V  ec=1.5  Tmeas=25 degC  Vge_vec=[ -2 6 7 8 10 12 15 20 ] V  Vce_vec=[ -1 0 0.5 1 1.5 2 2.5 3 3.5 4 ] V  T_vec=[25, 125] degC  Ic_mat=[ -1.015e-5 1.35e-8 4.7135e-4 5.092e-4 5.105e-4 5.117500000000001e-4 5.1299e-4 5.1423e-4 5.1548e-4 5.1672e-4; -9.986899999999999e-6 1.35e-8 4.7135e-4 5.092e-4 5.105e-4 5.117500000000001e-4 5.1299e-4 5.1423e-4 5.1548e-4 5.1672e-4; -9.955e-6 1.35e-8 0.0065225 3.3324 48.154 93.661 105.52 105.72 105.93 106.14; -9.955e-6 1.35e-8 0.0065235 3.5783 70.264 166.33 252.4 317.67 353.38 357.39; -9.955e-6 1.35e-8 0.006524 3.7206 89.17100000000001 228.09 371.63 511.02 642.6900000000001 764.04; -9.9549e-6 1.35e-8 0.0065242 3.7716 97.79300000000001 256.21 424.27 592.92 759.2 921.52; -9.9549e-6 1.35e-8 0.0065243 3.8067 104.52 278.11 464.6 654.37 844.5700000000001 1.0339e+3; -9.9549e-6 1.35e-8 0.0065244 3.8324 109.92 295.67 496.54 702.28 909.96 1.1183e+3 ] A  Ic_mat_3D=zeros(8, 10, 2) A  C_param=3  C_GE=23.7 nF  C_GC=2.7 nF  C_CE=0 nF  C_ies=9.85 nF  C_res=218 pF  C_oes=580 pF  C_GE_vec=[ 25 31 26.5 24.9 25 24.9 24.6 24.7 24.8 ] nF  C_GC_vec=[ 55 9 5.5 3.1 2.5 2.1 1.9 1.8 1.7 ] nF  C_CE_vec=[ 5 11 6.5 4.9 3.5 2.7 2.1 1.7 1.4 ] nF  C_ies_vec=[ 18 13 12 11 10 10 10 10 10 ] nF  C_res_vec=[ 6 2.7 1.9 1.3 0.36 0.22 0.19 0.17 0.16 ] nF  C_oes_vec=[ 8.5 4 3 2 0.8 0.6 0.5 0.48 0.43 ] nF  C_Vce_vec=[ 0 5 10 15 20 25 30 35 40 ] V  charge_linearity_param=1  C_OX=20 nF  V_C_OX=-5 V  TF=0 ns  VAF=10 V  RC=0.005 Ohm  RE=0.009 Ohm  RG=1 kOhm  BF=100  T_param=2  Ices_T2=1.5 mA  EG=0.0001 eV  Vce_sat_T2=2.45 V  Tmeas2=150 degC  XTI=1  BEX=-1  RG_alpha=1 1/K  Tdevice=150 degC  Tdevice_3D=25 degC  thermal_network_parameterization=ee.enum.thermalNetworkTopology.cauer  Rth=[0, 10] K/W  Rth_Foster=[4, 6] K/W  thermal_mass_parameterization=ee.enum.thermalNetwork.timeconstant  thermal_mass=[0, 1] J/K  thermal_mass_Foster=[1.5, 3] J/K  thermal_time_constant=[0, 10] s  thermal_time_constant_Foster=[6, 18] s  thermal_mass_initial_temperatures=[25, 25] degC  Ic_vec1=[0, 10, 50, 100, 200, 400, 600] A  Vce_vec1=[0, 1.1, 1.3, 1.45, 1.75, 2.25, 2.7] V  Rmiller=0.1 Ohm  Goff=1e-5 1/Ohm  t_on=0.07 us  t_rise=0.7 us  t_off=0.2 us  t_fall=0.5 us  v_meas=300 V  Tj_vec1=[298.15, 398.15] K  Vce_mat1=[0, 1.1, 1.3, 1.45, 1.75, 2.25, 2.7; 0, 1, 1.15, 1.35, 1.7, 2.35, 3] V  E_turn_on_mat1=[0, .2, 1, 2, 4, 8, 15; 0, .3, 1.3, 2.5, 5, 11, 18] * 1e-3 J  E_turn_off_mat1=[0, .3, 1.5, 3, 6, 15, 25; 0, .7, 3.3, 6.5, 13, 25, 35] * 1e-3 J
      settings: SourceProductName=Electrical  InternalSimscapePortConfiguration="{\"Bottom\":[],\"Left\":[{\"id\":\"G\",\"label\":\"\",\"type\":\"foundation.electrical.electrical\"}],\"Right\":[{\"id\":\"C\",\"label\":\"\",\"type\":\"foundation.electrical.electrical\"},{\"id\":\"E\",\"label\":\"\",\"type\":\"foundation.electrical.electrical\"}],\"Top\":[]}"
  N-Channel IGBT_C3-2 : ee_lib/Semiconductors & Converters/N-Channel IGBT  model_type=1  Ices=25 uA  Vces=1200 V  Vth=5 V  Vce_sat=2.25 V  Ice_sat=40 A  Vge_sat=7 V  ec=1.5  Tmeas=25 degC  Vge_vec=[ -2 6 7 8 10 12 15 20 ] V  Vce_vec=[ -1 0 0.5 1 1.5 2 2.5 3 3.5 4 ] V  T_vec=[25, 125] degC  Ic_mat=[ -1.015e-5 1.35e-8 4.7135e-4 5.092e-4 5.105e-4 5.117500000000001e-4 5.1299e-4 5.1423e-4 5.1548e-4 5.1672e-4; -9.986899999999999e-6 1.35e-8 4.7135e-4 5.092e-4 5.105e-4 5.117500000000001e-4 5.1299e-4 5.1423e-4 5.1548e-4 5.1672e-4; -9.955e-6 1.35e-8 0.0065225 3.3324 48.154 93.661 105.52 105.72 105.93 106.14; -9.955e-6 1.35e-8 0.0065235 3.5783 70.264 166.33 252.4 317.67 353.38 357.39; -9.955e-6 1.35e-8 0.006524 3.7206 89.17100000000001 228.09 371.63 511.02 642.6900000000001 764.04; -9.9549e-6 1.35e-8 0.0065242 3.7716 97.79300000000001 256.21 424.27 592.92 759.2 921.52; -9.9549e-6 1.35e-8 0.0065243 3.8067 104.52 278.11 464.6 654.37 844.5700000000001 1.0339e+3; -9.9549e-6 1.35e-8 0.0065244 3.8324 109.92 295.67 496.54 702.28 909.96 1.1183e+3 ] A  Ic_mat_3D=zeros(8, 10, 2) A  C_param=3  C_GE=23.7 nF  C_GC=2.7 nF  C_CE=0 nF  C_ies=9.85 nF  C_res=218 pF  C_oes=580 pF  C_GE_vec=[ 25 31 26.5 24.9 25 24.9 24.6 24.7 24.8 ] nF  C_GC_vec=[ 55 9 5.5 3.1 2.5 2.1 1.9 1.8 1.7 ] nF  C_CE_vec=[ 5 11 6.5 4.9 3.5 2.7 2.1 1.7 1.4 ] nF  C_ies_vec=[ 18 13 12 11 10 10 10 10 10 ] nF  C_res_vec=[ 6 2.7 1.9 1.3 0.36 0.22 0.19 0.17 0.16 ] nF  C_oes_vec=[ 8.5 4 3 2 0.8 0.6 0.5 0.48 0.43 ] nF  C_Vce_vec=[ 0 5 10 15 20 25 30 35 40 ] V  charge_linearity_param=1  C_OX=20 nF  V_C_OX=-5 V  TF=0 ns  VAF=10 V  RC=0.005 Ohm  RE=0.009 Ohm  RG=1 kOhm  BF=100  T_param=2  Ices_T2=1.5 mA  EG=0.0001 eV  Vce_sat_T2=2.45 V  Tmeas2=150 degC  XTI=1  BEX=-1  RG_alpha=1 1/K  Tdevice=150 degC  Tdevice_3D=25 degC  thermal_network_parameterization=ee.enum.thermalNetworkTopology.cauer  Rth=[0, 10] K/W  Rth_Foster=[4, 6] K/W  thermal_mass_parameterization=ee.enum.thermalNetwork.timeconstant  thermal_mass=[0, 1] J/K  thermal_mass_Foster=[1.5, 3] J/K  thermal_time_constant=[0, 10] s  thermal_time_constant_Foster=[6, 18] s  thermal_mass_initial_temperatures=[25, 25] degC  Ic_vec1=[0, 10, 50, 100, 200, 400, 600] A  Vce_vec1=[0, 1.1, 1.3, 1.45, 1.75, 2.25, 2.7] V  Rmiller=0.1 Ohm  Goff=1e-5 1/Ohm  t_on=0.07 us  t_rise=0.7 us  t_off=0.2 us  t_fall=0.5 us  v_meas=300 V  Tj_vec1=[298.15, 398.15] K  Vce_mat1=[0, 1.1, 1.3, 1.45, 1.75, 2.25, 2.7; 0, 1, 1.15, 1.35, 1.7, 2.35, 3] V  E_turn_on_mat1=[0, .2, 1, 2, 4, 8, 15; 0, .3, 1.3, 2.5, 5, 11, 18] * 1e-3 J  E_turn_off_mat1=[0, .3, 1.5, 3, 6, 15, 25; 0, .7, 3.3, 6.5, 13, 25, 35] * 1e-3 J
      settings: SourceProductName=Electrical  InternalSimscapePortConfiguration="{\"Bottom\":[],\"Left\":[{\"id\":\"G\",\"label\":\"\",\"type\":\"foundation.electrical.electrical\"}],\"Right\":[{\"id\":\"C\",\"label\":\"\",\"type\":\"foundation.electrical.electrical\"},{\"id\":\"E\",\"label\":\"\",\"type\":\"foundation.electrical.electrical\"}],\"Top\":[]}"
  to C3 : PMIOPort  Side=Left
  to A4 : PMIOPort  Port=2  Side=Left
  Phase : PMIOPort  Port=3  Side=Left
  Zero : PMIOPort  Port=4  Side=Right
  connections:
  N-Channel IGBT_A4/LConn1 -- to A4/RConn1
  Phase/RConn1 -- N-Channel IGBT_C3-2/RConn1 -- N-Channel IGBT_A4/RConn1 -- N-Channel IGBT_C3-1/RConn1
  Zero/RConn1 -- N-Channel IGBT_C3-1/RConn2 -- N-Channel IGBT_A4/RConn2 -- N-Channel IGBT_C3-2/RConn2
  N-Channel IGBT_C3-1/LConn1 -- to C3/RConn1 -- N-Channel IGBT_C3-2/LConn1

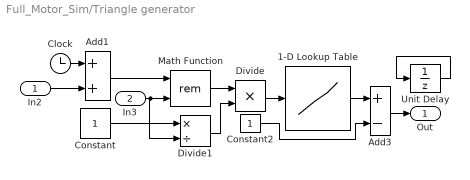
== system Full_Motor_Sim/Triangle generator ==
  In2 : Inport
  In3 : Inport  Port=2
  1-D Lookup Table : Lookup_n-D  NumberOfTableDimensions=1  BreakpointsForDimension1=[0 .5 1]  BeginIndexSearchUsingPreviousIndexResult=on  Table=[0 2 0]  InternalRulePriority=Speed  RndMeth=Simplest  InputSameDT=on
  Add1 : Sum
  Add3 : Sum  Inputs=+-
  Clock : Clock
  Constant : Constant
  Constant2 : Constant  SampleTime=0
  Divide : Product  Inputs=**
  Divide1 : Product  Inputs=*/
  Math Function : Math  Operator=rem  SignedPower=on  SaturateOnIntegerOverflow=on
  Unit Delay : UnitDelay  SampleTime=1e-5  HasFrameUpgradeWarning=on
  Out : Outport
  wires:
  Divide/1 -> 1-D Lookup Table/1
  Clock/1 -> Add1/1
  Unit Delay/1 -> Unit Delay/1
  In3/1 -> Divide1/2, Math Function/2
  In2/1 -> Add1/2
  Add3/1 -> Out/1
  Constant2/1 -> Add3/2
  1-D Lookup Table/1 -> Add3/1
  Add1/1 -> Math Function/1
  Math Function/1 -> Divide/1
  Divide1/1 -> Divide/2
  Constant/1 -> Divide1/1

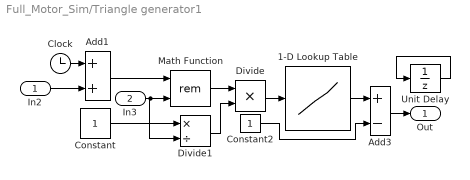
== system Full_Motor_Sim/Triangle generator1 ==
  In2 : Inport
  In3 : Inport  Port=2
  1-D Lookup Table : Lookup_n-D  NumberOfTableDimensions=1  BreakpointsForDimension1=[0 .5 1]  BeginIndexSearchUsingPreviousIndexResult=on  Table=[0 2 0]  InternalRulePriority=Speed  RndMeth=Simplest  InputSameDT=on
  Add1 : Sum
  Add3 : Sum  Inputs=+-
  Clock : Clock
  Constant : Constant
  Constant2 : Constant  SampleTime=0
  Divide : Product  Inputs=**
  Divide1 : Product  Inputs=*/
  Math Function : Math  Operator=rem  SignedPower=on  SaturateOnIntegerOverflow=on
  Unit Delay : UnitDelay  SampleTime=1e-5  HasFrameUpgradeWarning=on
  Out : Outport
  wires:
  Constant/1 -> Divide1/1
  Divide1/1 -> Divide/2
  Math Function/1 -> Divide/1
  Add1/1 -> Math Function/1
  1-D Lookup Table/1 -> Add3/1
  Constant2/1 -> Add3/2
  Add3/1 -> Out/1
  In2/1 -> Add1/2
  In3/1 -> Math Function/2, Divide1/2
  Unit Delay/1 -> Unit Delay/1
  Clock/1 -> Add1/1
  Divide/1 -> 1-D Lookup Table/1

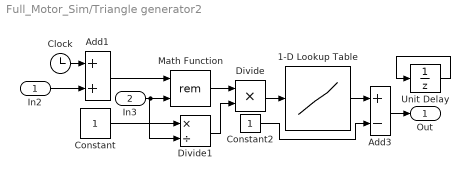
== system Full_Motor_Sim/Triangle generator2 ==
  In2 : Inport
  In3 : Inport  Port=2
  1-D Lookup Table : Lookup_n-D  NumberOfTableDimensions=1  BreakpointsForDimension1=[0 .5 1]  BeginIndexSearchUsingPreviousIndexResult=on  Table=[0 2 0]  InternalRulePriority=Speed  RndMeth=Simplest  InputSameDT=on
  Add1 : Sum
  Add3 : Sum  Inputs=+-
  Clock : Clock
  Constant : Constant
  Constant2 : Constant  SampleTime=0
  Divide : Product  Inputs=**
  Divide1 : Product  Inputs=*/
  Math Function : Math  Operator=rem  SignedPower=on  SaturateOnIntegerOverflow=on
  Unit Delay : UnitDelay  SampleTime=1e-5  HasFrameUpgradeWarning=on
  Out : Outport
  wires:
  Divide/1 -> 1-D Lookup Table/1
  Clock/1 -> Add1/1
  Unit Delay/1 -> Unit Delay/1
  In3/1 -> Divide1/2, Math Function/2
  In2/1 -> Add1/2
  Add3/1 -> Out/1
  Constant2/1 -> Add3/2
  1-D Lookup Table/1 -> Add3/1
  Add1/1 -> Math Function/1
  Math Function/1 -> Divide/1
  Divide1/1 -> Divide/2
  Constant/1 -> Divide1/1
